simulink model "validator"  (Simulink 7.6)
settings: Solver=ode15s  StartTime=0.0  StopTime=10.0  FixedStep=0.0001  RelTol=1e-3
libraries: fl_lib x17, nesl_utility x5, elec_lib x3
settings Model: Creator=Fodi  LastModifiedBy=Fodi

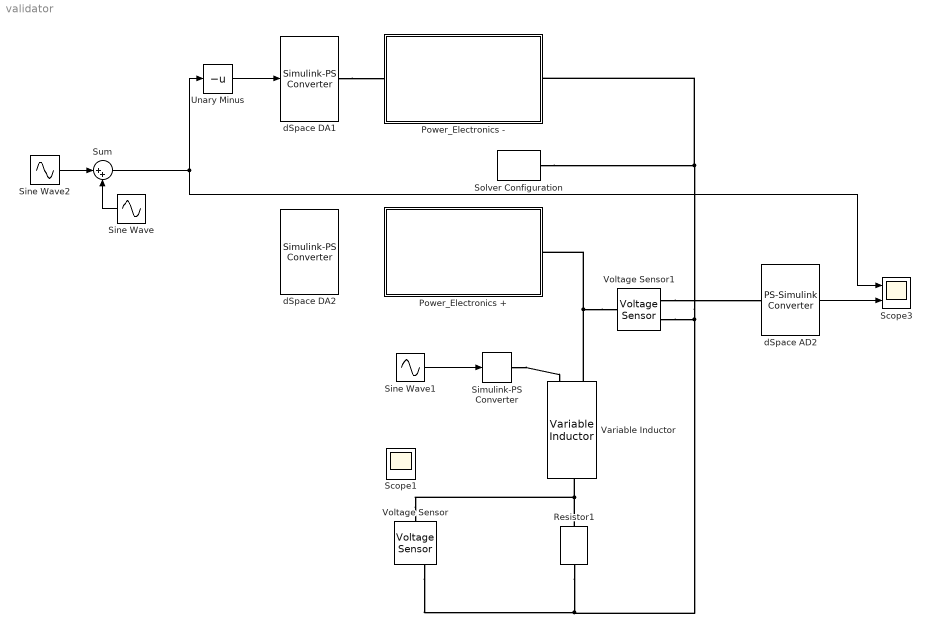
== system validator ==
  Power_Electronics + : Subsystem
  Power_Electronics - : Subsystem
  Resistor1 : fl_lib/Electrical/Electrical Elements/Resistor  DialogController=NetworkEngine.DynNeDlgSource  SystemSampleTime=-1  R=30 Ohm  i_Log=off  v_Log=off  LocalVarNames=|i|v  LocalVarDescs=|i|v  LocalVarLogging=[0 0]
  Scope1 : Scope
      settings: YMin=2.5065  YMax=2.513  SaveName=ScopeData5
  Scope3 : Scope  NumInputPorts=2
      settings: YMin=-0.00025~-0.05  YMax=0.00025~0.05  SaveName=ScopeData4
  Simulink-PS Converter : nesl_utility/Simulink-PS Converter  DialogController=NetworkEngine.DynNeUtilDlgSource  SystemSampleTime=-1  PhysicalDomain=network_engine_domain  LeftPortType=input  RightPortType=output  SubClassName=ps_input  Unit=1  AffineConversion=off  InputFilterTimeConstant=.001  UdotUserProvided=0
  Sine Wave : Sin  SineType=Sample based  SampleTime=0.0001
  Sine Wave1 : Sin  SineType=Sample based  Amplitude=1/1000  Bias=1  Samples=10000  SampleTime=0.0001
  Sine Wave2 : Sin  SineType=Sample based  Amplitude=0.1  Samples=1000  SampleTime=0.0001
  Solver Configuration : nesl_utility/Solver Configuration  DialogController=NetworkEngine.DynNeUtilDlgSource  SystemSampleTime=-1  PhysicalDomain=network_engine_domain  LeftPortType=input  RightPortType=generic  SubClassName=solver  Accelerate=off  Profile=off  ResidualTolerance=1e-9  MaxNonlinIter=3  MaxModeIter=2  DoFixedCost=off  UseLocalSampling=off  DoDC=off  LinearAlgebra=Sparse  LocalSolverSampleTime=.001  LocalSolverChoice=NE_BACKWARD_EULER_ADVANCER  UseLocalSolver=off
  Sum : Sum  Inputs=|++
  Unary Minus : UnaryMinus
  Variable Inductor : elec_lib/Passive Devices/Variable Inductor  DialogController=NetworkEngine.DynNeDlgSource  SystemSampleTime=-1  prm=2  Lmin=1e-6 H  g=1e-9 1/Ohm  i0=0 A  phi0=0 Wb  LocalVarLogging=[]
  Voltage Sensor : fl_lib/Electrical/Electrical Sensors/Voltage Sensor  DialogController=NetworkEngine.DynNeDlgSource  SystemSampleTime=-1  i1_Log=off  v1_Log=off  LocalVarNames=|i1|v1  LocalVarDescs=|i1|v1  LocalVarLogging=[0 0]
  Voltage Sensor1 : fl_lib/Electrical/Electrical Sensors/Voltage Sensor  DialogController=NetworkEngine.DynNeDlgSource  SystemSampleTime=-1  i1_Log=off  v1_Log=off  LocalVarNames=|i1|v1  LocalVarDescs=|i1|v1  LocalVarLogging=[0 0]
  dSpace AD2 : nesl_utility/PS-Simulink Converter  DialogController=NetworkEngine.DynNeUtilDlgSource  SystemSampleTime=-1  PhysicalDomain=network_engine_domain  LeftPortType=input  RightPortType=output  SubClassName=ps_output  Unit=1  AffineConversion=off
  dSpace DA1 : nesl_utility/Simulink-PS Converter  DialogController=NetworkEngine.DynNeUtilDlgSource  SystemSampleTime=-1  PhysicalDomain=network_engine_domain  LeftPortType=input  RightPortType=output  SubClassName=ps_input  Unit=1  AffineConversion=off  InputFilterTimeConstant=.001  UdotUserProvided=0
  dSpace DA2 : nesl_utility/Simulink-PS Converter  DialogController=NetworkEngine.DynNeUtilDlgSource  SystemSampleTime=-1  PhysicalDomain=network_engine_domain  LeftPortType=input  RightPortType=output  SubClassName=ps_input  Unit=1  AffineConversion=off  InputFilterTimeConstant=.001  UdotUserProvided=0
  wires:
  Unary Minus/1 -> dSpace DA1/1
  dSpace AD2/1 -> Scope3/2
  Sine Wave/1 -> Sum/2
  Sum/1 -> Unary Minus/1, Scope3/1
  Sine Wave1/1 -> Simulink-PS Converter/1
  Sine Wave2/1 -> Sum/1
  connections:
  Solver Configuration/RConn1 -- Voltage Sensor/RConn2 -- Resistor1/RConn1 -- Voltage Sensor1/RConn2 -- Power_Electronics -/RConn1
  Voltage Sensor1/LConn1 -- Variable Inductor/LConn2 -- Power_Electronics +/RConn1
  Voltage Sensor/LConn1 -- Resistor1/LConn1 -- Variable Inductor/RConn1
  Simulink-PS Converter/RConn1 -- Variable Inductor/LConn1
  dSpace DA1/RConn1 -- Power_Electronics -/LConn1
  Voltage Sensor1/RConn1 -- dSpace AD2/LConn1

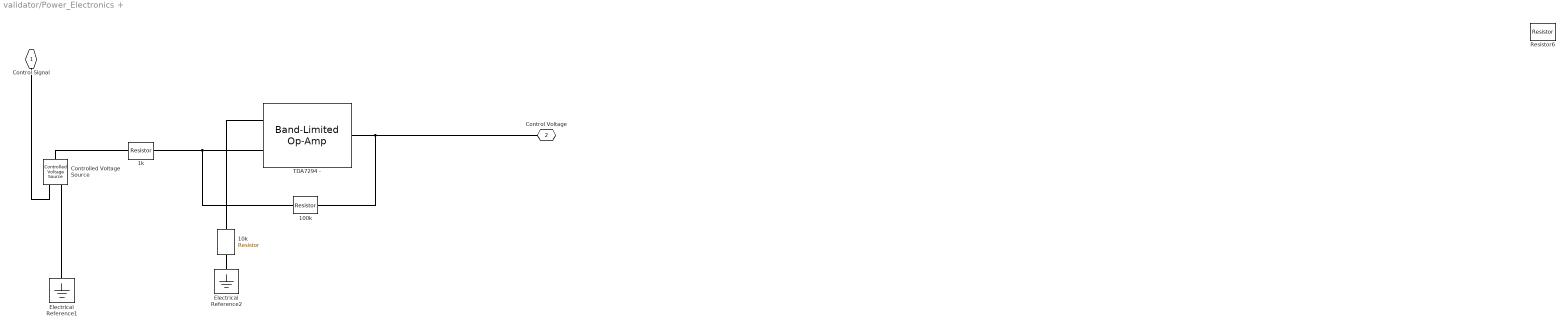
== system validator/Power_Electronics + ==
  100k : fl_lib/Electrical/Electrical Elements/Resistor  DialogController=NetworkEngine.DynNeDlgSource  SystemSampleTime=-1  R=10 kOhm  i_Log=off  v_Log=off  LocalVarNames=|i|v  LocalVarDescs=|i|v  LocalVarLogging=[0 0]
  10k : fl_lib/Electrical/Electrical Elements/Resistor  DialogController=NetworkEngine.DynNeDlgSource  SystemSampleTime=-1  R=100 kOhm  i_Log=off  v_Log=off  LocalVarNames=|i|v  LocalVarDescs=|i|v  LocalVarLogging=[0 0]
  1k : fl_lib/Electrical/Electrical Elements/Resistor  DialogController=NetworkEngine.DynNeDlgSource  SystemSampleTime=-1  R=100 Ohm  i_Log=off  v_Log=off  LocalVarNames=|i|v  LocalVarDescs=|i|v  LocalVarLogging=[0 0]
  Controlled Voltage Source : fl_lib/Electrical/Electrical Sources/Controlled Voltage Source  DialogController=NetworkEngine.DynNeDlgSource  SystemSampleTime=-1  i_Log=off  v_Log=off  LocalVarNames=|i|v  LocalVarDescs=|i|v  LocalVarLogging=[0 0]
  Electrical Reference1 : fl_lib/Electrical/Electrical Elements/Electrical Reference  DialogController=NetworkEngine.DynNeDlgSource  SystemSampleTime=-1  i_Log=off  LocalVarNames=|i  LocalVarDescs=|i  LocalVarLogging=0
  Electrical Reference2 : fl_lib/Electrical/Electrical Elements/Electrical Reference  DialogController=NetworkEngine.DynNeDlgSource  SystemSampleTime=-1  i_Log=off  LocalVarNames=|i  LocalVarDescs=|i  LocalVarLogging=0
  Resistor6 : fl_lib/Electrical/Electrical Elements/Resistor  DialogController=NetworkEngine.DynNeDlgSource  SystemSampleTime=-1  R=1 kOhm  i_Log=off  v_Log=off  LocalVarNames=|i|v  LocalVarDescs=|i|v  LocalVarLogging=[0 0]
  TDA7294 - : elec_lib/Integrated Circuits/Band-Limited Op-Amp  DialogController=NetworkEngine.DynNeDlgSource  SystemSampleTime=-1  A=10000  Rin=100 kOhm  Rout=100 Ohm  Vmin=-35 V  Vmax=35 V  Vdotmax=7000000 V/s  f=1e+5 Hz  V0=0 V  LocalVarLogging=[]
  Control Signal : PMIOPort  Tag=PMCPort  Port=1  Side=Left
  Control Voltage : PMIOPort  Tag=PMCPort  Port=2  Side=Right
  connections:
  1k/RConn1 -- TDA7294 -/LConn2 -- 100k/LConn1
  Electrical Reference1/LConn1 -- Controlled Voltage Source/RConn2
  Control Signal/RConn1 -- Controlled Voltage Source/RConn1
  10k/RConn1 -- Electrical Reference2/LConn1
  Control Voltage/RConn1 -- TDA7294 -/RConn1 -- 100k/RConn1
  TDA7294 -/LConn1 -- 10k/LConn1
  Controlled Voltage Source/LConn1 -- 1k/LConn1

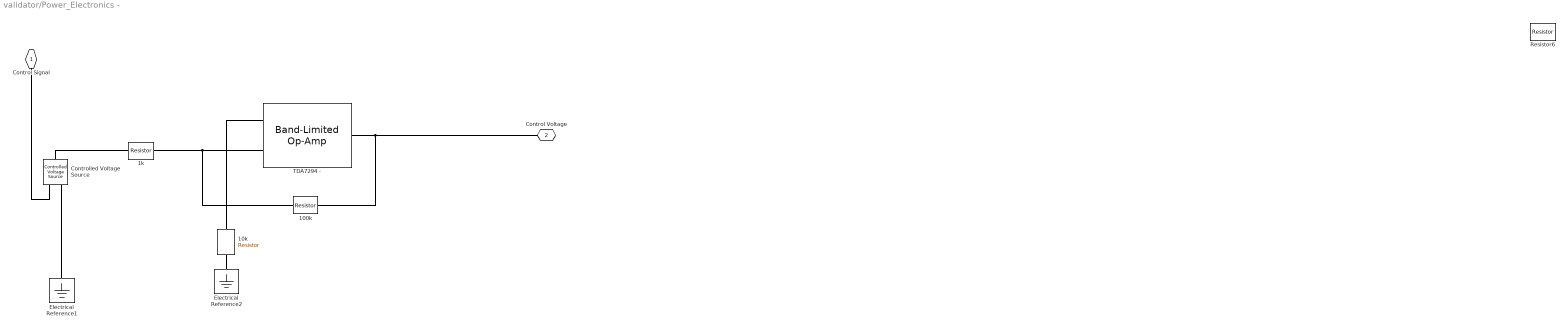
== system validator/Power_Electronics - ==
  100k : fl_lib/Electrical/Electrical Elements/Resistor  DialogController=NetworkEngine.DynNeDlgSource  SystemSampleTime=-1  R=100 kOhm  i_Log=off  v_Log=off  LocalVarNames=|i|v  LocalVarDescs=|i|v  LocalVarLogging=[0 0]
  10k : fl_lib/Electrical/Electrical Elements/Resistor  DialogController=NetworkEngine.DynNeDlgSource  SystemSampleTime=-1  R=10 kOhm  i_Log=off  v_Log=off  LocalVarNames=|i|v  LocalVarDescs=|i|v  LocalVarLogging=[0 0]
  1k : fl_lib/Electrical/Electrical Elements/Resistor  DialogController=NetworkEngine.DynNeDlgSource  SystemSampleTime=-1  R=1 kOhm  i_Log=off  v_Log=off  LocalVarNames=|i|v  LocalVarDescs=|i|v  LocalVarLogging=[0 0]
  Controlled Voltage Source : fl_lib/Electrical/Electrical Sources/Controlled Voltage Source  DialogController=NetworkEngine.DynNeDlgSource  SystemSampleTime=-1  i_Log=off  v_Log=off  LocalVarNames=|i|v  LocalVarDescs=|i|v  LocalVarLogging=[0 0]
  Electrical Reference1 : fl_lib/Electrical/Electrical Elements/Electrical Reference  DialogController=NetworkEngine.DynNeDlgSource  SystemSampleTime=-1  i_Log=off  LocalVarNames=|i  LocalVarDescs=|i  LocalVarLogging=0
  Electrical Reference2 : fl_lib/Electrical/Electrical Elements/Electrical Reference  DialogController=NetworkEngine.DynNeDlgSource  SystemSampleTime=-1  i_Log=off  LocalVarNames=|i  LocalVarDescs=|i  LocalVarLogging=0
  Resistor6 : fl_lib/Electrical/Electrical Elements/Resistor  DialogController=NetworkEngine.DynNeDlgSource  SystemSampleTime=-1  R=1 kOhm  i_Log=off  v_Log=off  LocalVarNames=|i|v  LocalVarDescs=|i|v  LocalVarLogging=[0 0]
  TDA7294 - : elec_lib/Integrated Circuits/Band-Limited Op-Amp  DialogController=NetworkEngine.DynNeDlgSource  SystemSampleTime=-1  A=10000  Rin=100 kOhm  Rout=100 Ohm  Vmin=-35 V  Vmax=35 V  Vdotmax=7000000 V/s  f=1e+5 Hz  V0=0 V  LocalVarLogging=[]
  Control Signal : PMIOPort  Tag=PMCPort  Port=1  Side=Left
  Control Voltage : PMIOPort  Tag=PMCPort  Port=2  Side=Right
  connections:
  Controlled Voltage Source/LConn1 -- 1k/LConn1
  TDA7294 -/LConn1 -- 10k/LConn1
  Control Voltage/RConn1 -- 100k/RConn1 -- TDA7294 -/RConn1
  10k/RConn1 -- Electrical Reference2/LConn1
  Control Signal/RConn1 -- Controlled Voltage Source/RConn1
  Electrical Reference1/LConn1 -- Controlled Voltage Source/RConn2
  100k/LConn1 -- TDA7294 -/LConn2 -- 1k/RConn1
